simulink model "prioritydemo"  (R2017b)
settings: Solver=VariableStepDiscrete  StartTime=0.0  StopTime=inf  RelTol=1e-3  EnableMultiTasking=on
undefined symbols (not defined in the file or in its folder): gcbh
Description:
  | Block Priority
  | 
  | This model shows what happens when blocks are assigned different
  | priorities.  The block priority affects the order in which the blocks are
  | executed.  You can set the block priority through the Block Properties dialog.
  | 
  | The block sorting order is calculated only at the beginning of a
  | simulation.  For this reason, changes to a block's Priority property are only
  | updated when the simulation is started.  Double click on the green block
  | to change the priority levels for the blocks and see what happens.
  | 
  | Inside of each triggered subsystem is an S-Function which controls the coloring
  | of the blocks and also slows down the simulation. The priority level of the block
  | is displayed using the format attribute string that can be set in the Block Properties
  | dialog.
settings Model: ExtModeTrigMode=oneshot  ExtModeArmWhenConnect=off  ExtModeAutoUpdateStatusClock=off  Creator=The MathWorks, Inc.  LastModifiedBy=prave
settings DataIOCC: SaveFormat=Array
settings OptimizationCC: BlockReduction=off  BooleanDataType=off  ExpressionDepthLimit=2147483647  InitFltsAndDblsToZero=on  LifeSpan=inf  BufferReusableBoundary=off
settings DebuggingCC: SaveWithParameterizedLinksMsg=none  UnderspecifiedInitializationDetection=Classic  MergeDetectMultiDrivingBlocksExec=none  SignalResolutionControl=TryResolveAllWithWarning  MultiTaskDSMMsg=warning  MultiTaskCondExecSysMsg=none  IntegerOverflowMsg=none  FcnCallInpInsideContextMsg=warning  BusObjectLabelMismatch=none  AllowSymbolicDim=off  StateNameClashWarn=warning  SFUnexpectedBacktrackingDiag=warning  SFNoUnconditionalDefaultTransitionDiag=warning  SFExecutionAtInitializationDiag=none  IntegerSaturationMsg=none
settings HardwareCC: ProdBitPerPointer=32  ProdBitPerSizeT=32  ProdBitPerPtrDiffT=32  ProdLargestAtomicFloat=None  ProdIntDivRoundTo=Undefined  ProdEndianess=Unspecified  ProdWordSize=32  ProdHWDeviceType=32-bit Generic  TargetUnknown=on
settings ModelReferenceCC: PropagateSignalLabelsOutOfModel=off
settings RTWCC: Description=Generic Real-Time Target
settings CodeAppCC: StateflowObjectComments=on
settings GRTTargetCC: TargetFcnLib=ansi_tfl_tmw.mat  TargetLangStandard=C89/C90 (ANSI)  GeneratePreprocessorConditionals=Disable all  CombineOutputUpdateFcns=off  GRTInterface=on
settings ConfigComp: CovMetricSettings=dw  CovHtmlReporting=on  CovSaveCumulativeToWorkspaceVar=on  CovSaveSingleToWorkspaceVar=on  CovExternalEMLEnable=off

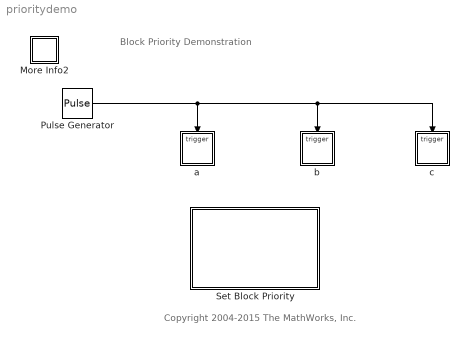
== system prioritydemo ==
  note: Block Priority Demonstration
  note: Copyright 2004-2015 The MathWorks, Inc.
  More Info2 : Subsystem
      settings: OpenFcn=showdemo(bdroot(gcs))
      mask Display: disp('?')
  Pulse Generator : DiscretePulseGenerator
  Set Block Priority : Subsystem  StartFcn=set_param(gcbh,'MaskEnables',{'off'})  StopFcn=set_param(gcbh,'MaskEnables',{'on'})  mask(Set Block Priority){PriorityOrder=1 2 3}
      mask prompts: PriorityOrder "Priority order:"
      mask help: This block lets you select the priority that is used on the three triggered subsystems above it. The priority may only be set when the simulation is stopped.
      mask init:
      | spriorityfcn([],[],[],'PriorityOrder');
      mask TypeOptions PriorityOrder: 1 2 3 | 1 3 2 | 2 1 3 | 2 3 1 | 3 1 2 | 3 2 1
      mask Display: disp(['Set\nBlock\nPriority\n' PriorityOrder])
  a : Subsystem  Priority=1
      settings: AttributesFormatString=Priority: %<Priority>
  b : Subsystem  Priority=2
      settings: AttributesFormatString=Priority: %<Priority>
  c : Subsystem  Priority=3
      settings: AttributesFormatString=Priority: %<Priority>
  wires:
  Pulse Generator/1 -> c/Trigger, b/Trigger, a/Trigger

== system prioritydemo/More Info2 ==

== system prioritydemo/Set Block Priority ==

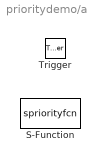
== system prioritydemo/a ==
  Trigger : TriggerPort  VariantControl=(inherit)
  S-Function : S-Function  FunctionName=spriorityfcn  SFunctionDeploymentMode=off  EnableBusSupport=off

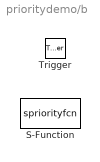
== system prioritydemo/b ==
  Trigger : TriggerPort  VariantControl=(inherit)
  S-Function : S-Function  FunctionName=spriorityfcn  SFunctionDeploymentMode=off  EnableBusSupport=off

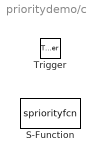
== system prioritydemo/c ==
  Trigger : TriggerPort  VariantControl=(inherit)
  S-Function : S-Function  FunctionName=spriorityfcn  SFunctionDeploymentMode=off  EnableBusSupport=off
